simulink model "DPSK_RX"  (R2018a)
settings: Solver=VariableStepAuto  StartTime=0.0  StopTime=inf  RelTol=1e-3
values from neighbouring files (symbols this model uses):
  sdrqpskrx =     [sdrqpskrx.mat]
libraries: commsync2 x3, commrfcorlib x2, dspstat3 x2, commdigbbndpm3 x2, commutil2 x2, sdrublksprivate x1, commrflib2 x1, dspsigops x1, commsequence2 x1, commsink2 x1, dspsrcs4 x1, commfilt2 x1
settings Model: Creator=n53s123  LastModifiedBy=n53s123

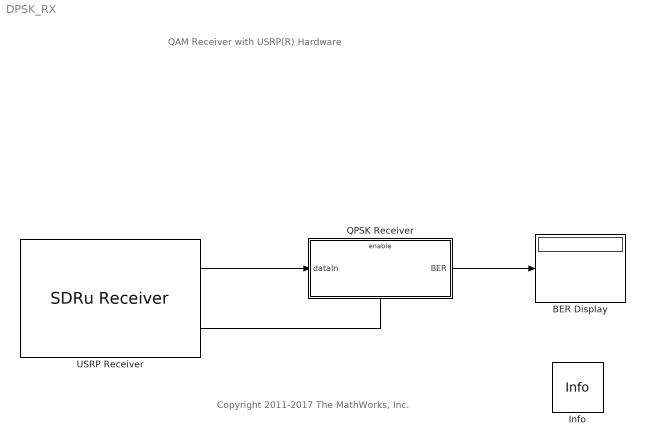
== system DPSK_RX ==
  note: Copyright 2011-2017 The MathWorks, Inc.
  note: QAM Receiver with USRP(R) Hardware
  BER Display : Display
  Info : sdrublksprivate/Info  SystemSampleTime=-1
      settings: SourceProductName=Communications System Toolbox Support Package for USRP(R) Radio  SourceProductBaseCode=USRP
  QPSK Receiver : Subsystem
      mask Display: disp('QAM Receiver')
  USRP Receiver : commsdrhw_v2/SDRu Receiver  SourceLibraryInfo="This block requires <a href=\"http://www.mathworks.com/hardware-support/usrp.html\">Communications System Toolbox Support Package for USRP Radio</a>"  rxtx=rx  initializeIPAddress=0  devMap=0  USRP2_IP=192.168.10.2  USRP_IP_X300=192.168.10.2  USRP_IP_X310=192.168.10.2  USRP_serialNumB200=30B2ACA  USRP_serialNumB210=ECR04ZDBT  platform=N200/N210/USRP2  prevPlatform=N200/N210/USRP2  lastIPAddressPopup=192.168.10.2  USRP_ID=192.168.10.2  LastIPAddress=192.168.10.2  ChannelMapping=1  centerFrequencySrc=Dialog  centerFrequency=15000000  loOffsetSrc=Dialog  loOffset=0  gainSrc=Dialog  gain=0  PPSSource=Internal  clockSource=Internal  masterClkRateParam=100e6  masterClkRateB200=sdrqpskrx.MasterClockRate  masterClkRateB210=sdrqpskrx.MasterClockRate  masterClkRateX300=200e6  masterClkRateX310=200e6  masterClkRate=100e6  decimInterpSrc=Dialog  decimInterp=sdrqpskrx.USRPDecimationFactor  USRP2_IP_NUM=[49 57 50 46 49 54 56 46 49 48 46 50]  TransportDataType=int16  overrunUnderrunPort=off  sampleTime=1/sdrqpskrx.USRPFrontEndSampleRate  outputDatatype=double  frameLength=sdrqpskrx.USRPFrameLength  HOST_DATA_PORT=0  HOST_CONTROL_PORT=0  USRP2_DATA_PORT=0  USRP2_CONTROL_PORT=0  bufferMode=Continuous streaming  EnableBurstMode=off  NumFramesInBurst=100
      settings: SourceProductName=Communications System Toolbox Support Package for USRP(R) Radio  SourceProductBaseCode=USRP
  wires:
  QPSK Receiver/1(BER) -> BER Display/1
  USRP Receiver/2 -> QPSK Receiver/Enable
  USRP Receiver/1 -> QPSK Receiver/1(dataIn)

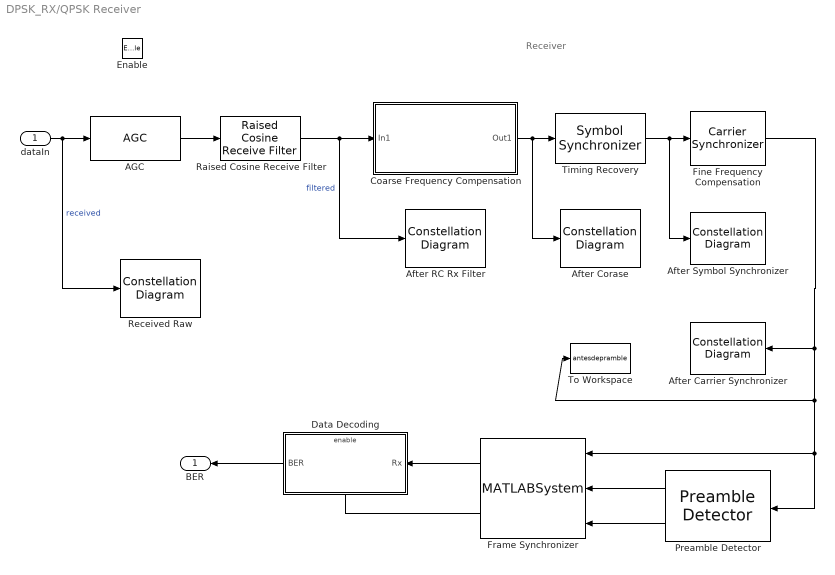
== system DPSK_RX/QPSK Receiver ==
  note: Receiver
  dataIn : Inport
  Enable : EnablePort  PropagateVarSize=During execution
  AGC : commrfcorlib/AGC  LegacyMode=off  DetectorMethod=Rectifier  LoopMethod=Linear  UpdatePeriod=100  StepSize=0.1  AdaptationStepSize=0.01  DesiredOutputPower=sdrqpskrx.DesiredPower  AveragingLength=sdrqpskrx.AveragingLength  MaximumGain=30  MaxPowerGain=sdrqpskrx.MaxPowerGain  GainOutputPort=off  InputPowerOutputPort=off  SimulateUsing=Code generation
      settings: SourceProductName=Communications System Toolbox
  After Carrier Synchronizer : ConstellationDiagram  Tag=ScatterPlot
  After Corase : ConstellationDiagram  Tag=ScatterPlot
  After RC Rx Filter : ConstellationDiagram  Tag=ScatterPlot
  After Symbol Synchronizer : ConstellationDiagram  Tag=ScatterPlot
  Coarse Frequency Compensation : Subsystem
      mask Display: fprintf('Coarse Frequency\nCompensation')
  Data Decoding : Subsystem
      mask Display: disp('Data Decoding');
  Fine Frequency Compensation : commsync2/Carrier Synchronizer  Modulation=QPSK  ModulationPhaseOffset=Auto  CustomPhaseOffset=0  SamplesPerSymbol=sdrqpskrx.Interpolation/sdrqpskrx.Decimation  DampingFactor=1  NormalizedLoopBandwidth=0.01  EstimatedPhaseErrorOutputPort=off  SimulateUsing=Code generation
      settings: SourceProductName=Communications System Toolbox
  Frame Synchronizer : MATLABSystem  System=FrameSynchronizer  Input=Symbol  OutputFrameLength=sdrqpskrx.FrameSize  PreambleLength=sdrqpskrx.BarkerLength  SimulateUsing=Code generation
      mask Type: FrameSynchronizer
      mask Display:
      | disp(['Frame' char(10) 'Synchronizer']);
      | port_label('input',1,'u');
      | port_label('input',2,'idx');
      | port_label('input',3,'dtMt');
      | port_label('output',1,'Frame');
      | port_label('output',2,'Valid');
  Preamble Detector : commsync2/Preamble Detector  Input=Symbol  Preamble=Barker  Threshold=10.5  DetectionMetricOutput=on  Detections=All  SimulateUsing=Code generation
      settings: SourceProductName=Communications System Toolbox  SourceProductBaseCode=CM
  Raised Cosine Receive Filter : commfilt2/Raised Cosine Receive Filter  filtType=Square root  R=sdrqpskrx.RolloffFactor  filtSpan=sdrqpskrx.RaisedCosineFilterSpan  N=sdrqpskrx.Interpolation  downFactor=sdrqpskrx.Decimation  downOffset=0  filterGain=1  InputProcessing=Columns as channels (frame based)  RateOptions=Enforce single-rate processing  framing=Mute  checkCoeff=off  variableName=rcRxFilt  currentFiltSpan=10  D=5  inputOffset=0  sampMode=Mute  saveAsFlag=0  rateMode=Downsampling  checkGain=Normalized  launchFVT=on  roundingMode=Floor  overflowMode=off  coeffDataTypeStr=Inherit: Same word length as input  coeffMin=[]  coeffMax=[]  coeffLastDataTypeStr=Inherit: Same word length as input  accumDataTypeStr=Inherit: Same as product output  accumLastDataTypeStr=Inherit: Same as product output  outputDataTypeStr=Inherit: Same as accumulator  outputMin=[]  outputMax=[]  outputLastDataTypeStr=Inherit: Same as accumulator
  Received Raw : ConstellationDiagram  Tag=ScatterPlot
  Timing Recovery : commsync2/Symbol Synchronizer  Modulation=PAM/PSK/QAM  TimingErrorDetector=Gardner (non-data-aided)  SamplesPerSymbol=2  DampingFactor=1  NormalizedLoopBandwidth=0.01  DetectorGain=sdrqpskrx.TimingErrorDetectorGain  TimingErrorOutputPort=off  SimulateUsing=Code generation
      settings: SourceProductName=Communications System Toolbox  SourceProductBaseCode=CM
  To Workspace : ToWorkspace  VariableName=antesdepramble  SaveFormat=Structure With Time  SampleTime=-1
  BER : Outport
  wires:
  Raised Cosine Receive Filter/1 -> Coarse Frequency Compensation/1(In1), After RC Rx Filter/1  "filtered"
  Preamble Detector/2 -> Frame Synchronizer/3
  Frame Synchronizer/2 -> Data Decoding/Enable
  Preamble Detector/1 -> Frame Synchronizer/2
  Frame Synchronizer/1 -> Data Decoding/1(Rx)
  Coarse Frequency Compensation/1(Out1) -> After Corase/1, Timing Recovery/1
  Data Decoding/1(BER) -> BER/1
  AGC/1 -> Raised Cosine Receive Filter/1
  Fine Frequency Compensation/1 -> To Workspace/1, Frame Synchronizer/1, Preamble Detector/1, After Carrier Synchronizer/1
  Timing Recovery/1 -> Fine Frequency Compensation/1, After Symbol Synchronizer/1
  dataIn/1 -> Received Raw/1, AGC/1  "received"

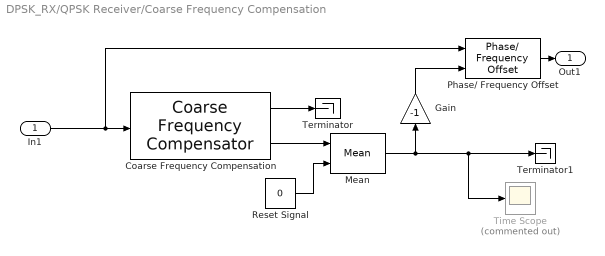
== system DPSK_RX/QPSK Receiver/Coarse Frequency Compensation ==
  In1 : Inport
  Coarse Frequency Compensation : commrfcorlib/Coarse Frequency Compensator  Modulation=QPSK  Algorithm=Correlation-based  FrequencyResolution=25  MaximumFrequencyOffset=12.5e3  SamplesPerSymbol=4  EstimatedFreqOffsetPort=on  SimulateUsing=Code generation
      settings: SourceProductName=Communications System Toolbox  SourceProductBaseCode=CM
  Gain : Gain  Gain=-1
  Mean : dspstat3/Mean  run=on  InputProcessing=Columns as channels (frame based)  reset_popup=Either edge  directionMode=Each column  dimension=1  roiEnable=off  roiType=Rectangles  roiPortion=Entire ROI  roiOutput=Individual statistics for each ROI  roiFlag=off  roundingMode=Floor  overflowMode=off  outputDataTypeStr=Inherit: Same as accumulator  outputMin=[]  outputMax=[]  outputLastDataTypeStr=Inherit: Same as accumulator
  Phase/ Frequency Offset : commrflib2/Phase// Frequency Offset  phaseOffset=0  freqPort=on  freqOffset=0
      settings: SourceProductName=Communications System Toolbox
  Reset Signal : Constant  Value=0
  Terminator : Terminator
  Terminator1 : Terminator
  Time Scope : Scope  Commented=on
  Out1 : Outport
  wires:
  In1/1 -> Phase/ Frequency Offset/1, Coarse Frequency Compensation/1
  Phase/ Frequency Offset/1 -> Out1/1
  Mean/1 -> Time Scope/1, Terminator1/1, Gain/1
  Coarse Frequency Compensation/2 -> Mean/1
  Coarse Frequency Compensation/1 -> Terminator/1
  Gain/1 -> Phase/ Frequency Offset/2
  Reset Signal/1 -> Mean/2

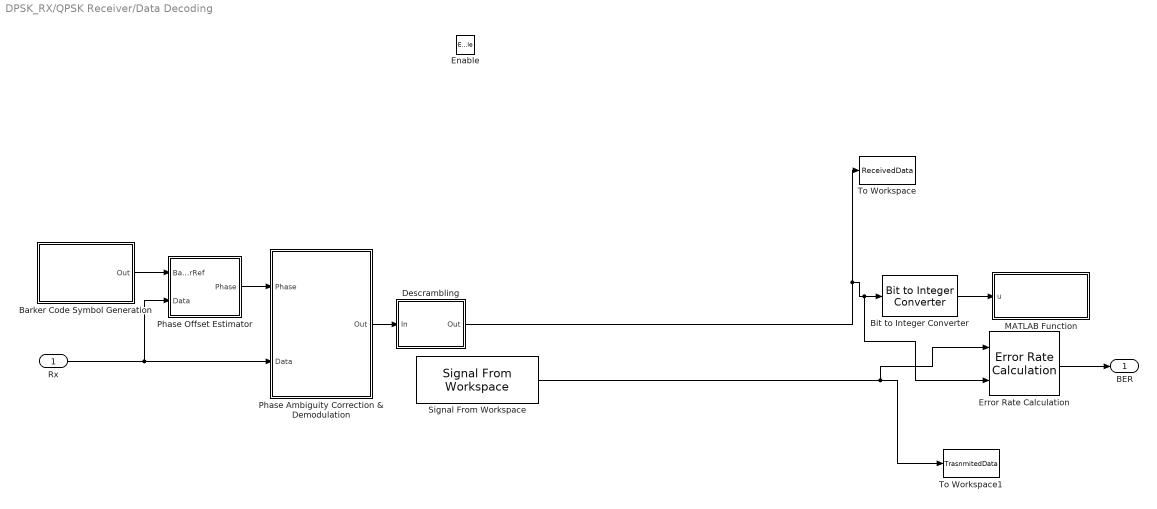
== system DPSK_RX/QPSK Receiver/Data Decoding ==
  Rx : Inport
  Enable : EnablePort
  "Barker Code Symbol Generation " : Subsystem
      mask Display: disp('Barker Code\nSymbol Generation')
  Bit to Integer Converter : commutil2/Bit to Integer Converter  nbits=7  bitOrder=MSB first  signedOutputValues=Unsigned  outDtype=Inherit via internal rule  outDtypeSigned=Inherit via internal rule
  Descrambling : Subsystem
      mask Display: disp('Descrambling');
  Error Rate Calculation : commsink2/Error Rate Calculation  N=0  st_delay=0  cp_mode=Select samples from mask  subframe=sdrqpskrx.BerMask  PMode=Port  WsName=ErrorVec  RsMode2=off  stop=off  numErr=100  maxBits=1e6
  MATLAB Function : MATLAB Function  TreatAsAtomicUnit=on
  Phase Ambiguity Correction & Demodulation : Subsystem
      mask Display: disp('Phase Ambiguity\nCorrection\n& Demodulation');
  Phase Offset Estimator : Subsystem
  Signal From Workspace : dspsrcs4/Signal From Workspace  X=sdrqpskrx.MessageBits  Ts=1/sdrqpskrx.PayloadLength*sdrqpskrx.FrameTime  nsamps=sdrqpskrx.MessageLength * 7 * sdrqpskrx.NumberOfMessage  OutputAfterFinalValue=Cyclic repetition  ignoreOrWarnInputAndFrameLengths=off  OutputFrames=off
  To Workspace : ToWorkspace  VariableName=ReceivedData  SampleTime=-1
  To Workspace1 : ToWorkspace  VariableName=TrasnmitedData  SampleTime=-1
  BER : Outport
  wires:
  "Barker Code Symbol Generation "/1(Out) -> Phase Offset Estimator/1(BarkerRef)
  Phase Offset Estimator/1(Phase) -> Phase Ambiguity Correction & Demodulation/1(Phase)
  Rx/1 -> Phase Offset Estimator/2(Data), Phase Ambiguity Correction & Demodulation/2(Data)
  Error Rate Calculation/1 -> BER/1
  Phase Ambiguity Correction & Demodulation/1(Out) -> Descrambling/1(In)
  Signal From Workspace/1 -> Error Rate Calculation/1, To Workspace1/1
  Bit to Integer Converter/1 -> MATLAB Function/1(u)
  Descrambling/1(Out) -> Error Rate Calculation/2, Bit to Integer Converter/1, To Workspace/1

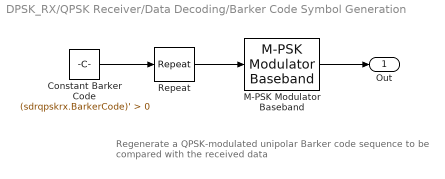
== system DPSK_RX/QPSK Receiver/Data Decoding/Barker Code Symbol Generation  ==
  note: Regenerate a QPSK-modulated unipolar Barker code sequence
      | to be compared with the received data
  Constant Barker Code : Constant  Value=(sdrqpskrx.BarkerCode)' > 0  VectorParams1D=off  OutDataTypeStr=double
  M-PSK Modulator Baseband : commdigbbndpm3/M-PSK Modulator Baseband  M=16  InType=Bit  Enc=Gray  Mapping=[0:7]  Ph=0  outDtype=double  outWordLen=16  outUDDataType=sfix(16)  outFracLenMode=Best precision  outFracLen=15  outDataTypeStr=double  outLastDataTypeStr=double
      settings: SourceProductName=Communications System Toolbox
  Repeat : dspsigops/Repeat  N=4  InputProcessing=Columns as channels (frame based)  RateOptions=Enforce single-rate processing  ic=0  mode=Unused parameter value
      settings: SourceProductName=DSP System Toolbox
  Out : Outport
  wires:
  Constant Barker Code/1 -> Repeat/1
  Repeat/1 -> M-PSK Modulator Baseband/1
  M-PSK Modulator Baseband/1 -> Out/1

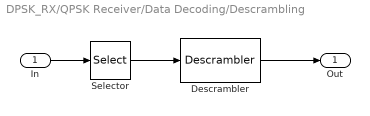
== system DPSK_RX/QPSK Receiver/Data Decoding/Descrambling ==
  In : Inport
  Descrambler : commsequence2/Descrambler  M=2  poly=[1 1 1 0 1]  iniStaSource=Dialog Parameter  ini_sta=[0 0 0 0]  resetViaPort=off
      settings: SourceProductName=Communications System Toolbox  SourceProductBaseCode=CM
  Selector : Selector  IndexOptions=Index vector (dialog)  Indices=[sdrqpskrx.HeaderLength+(1 : sdrqpskrx.PayloadLength)]  OutputSizes=1
  Out : Outport
  wires:
  In/1 -> Selector/1
  Selector/1 -> Descrambler/1
  Descrambler/1 -> Out/1

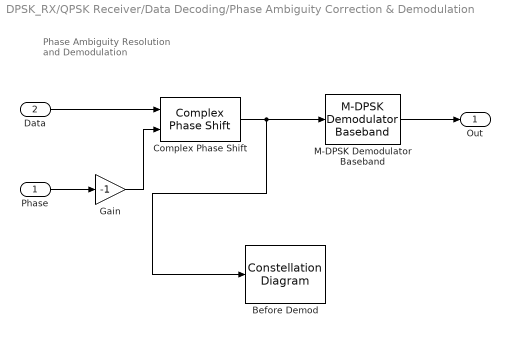
== system DPSK_RX/QPSK Receiver/Data Decoding/Phase Ambiguity Correction & Demodulation ==
  note: Phase Ambiguity Resolution
      | and Demodulation
  Phase : Inport
  Data : Inport  Port=2
  "Before Demod " : ConstellationDiagram  Tag=ScatterPlot
  Complex Phase Shift : commutil2/Complex Phase Shift
      settings: SourceProductName=Communications System Toolbox  SourceProductBaseCode=CM
  Gain : Gain  Gain=-1  OutDataTypeStr=Inherit: Same as input
  M-DPSK Demodulator Baseband : commdigbbndpm3/M-DPSK Demodulator Baseband  M=16  OutType=Bit  Dec=Gray  Ph=0  outDtype1=Inherit via internal rule  outDtype2=Inherit via internal rule
      settings: SourceProductName=Communications System Toolbox  SourceProductBaseCode=CM
  Out : Outport
  wires:
  Phase/1 -> Gain/1
  M-DPSK Demodulator Baseband/1 -> Out/1
  Data/1 -> Complex Phase Shift/1
  Gain/1 -> Complex Phase Shift/2
  Complex Phase Shift/1 -> M-DPSK Demodulator Baseband/1, "Before Demod "/1

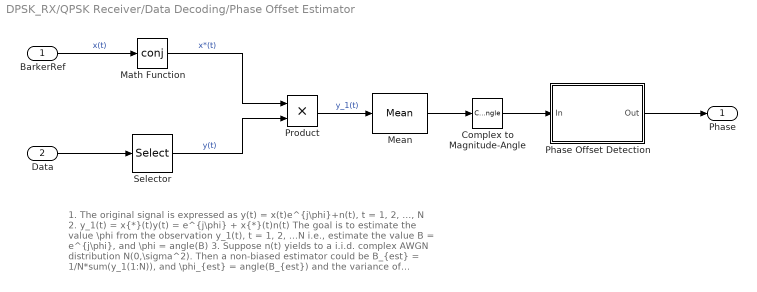
== system DPSK_RX/QPSK Receiver/Data Decoding/Phase Offset Estimator ==
  note: 1. The original signal is expressed as y(t) = x(t)e^{j\phi}+n(t), t = 1, 2, ..., N
      | 2. y_1(t) = x{*}(t)y(t) = e^{j\phi} + x{*}(t)n(t)
      | The goal is to estimate the value \phi from the observation y_1(t), t = 1, 2, ...N
      | i.e., estimate the value B = e^{j\phi}, and \phi = angle(B)
      | 3. Suppose n(t) yields to a i.i.d. complex AWGN distribution N(0,\sigma^2).
      | Then a non-biased estimator could be
      | B_{est} = 1/N*sum(y_1(1:N)), and \phi_{est} = angle(B_{est})
      | and the variance of B_{est} is \sigma^2/N
  BarkerRef : Inport
  Data : Inport  Port=2
  Complex to Magnitude-Angle : ComplexToMagnitudeAngle  Output=Angle
  Math Function : Math  Operator=conj  SaturateOnIntegerOverflow=on
  Mean : dspstat3/Mean  run=off  InputProcessing=Columns as channels (frame based)  reset_popup=None  directionMode=Each column  dimension=1  roiEnable=off  roiType=Rectangles  roiPortion=Entire ROI  roiOutput=Individual statistics for each ROI  roiFlag=off  roundingMode=Floor  overflowMode=off  outputDataTypeStr=Inherit: Same as accumulator  outputMin=[]  outputMax=[]  outputLastDataTypeStr=Inherit: Same as accumulator
  Phase Offset Detection : MATLAB Function  TreatAsAtomicUnit=on
  Product : Product  RndMeth=Zero
  Selector : Selector  IndexOptions=Index vector (dialog)  Indices=[1:sdrqpskrx.BarkerLength]  OutputSizes=1
  Phase : Outport
  wires:
  Data/1 -> Selector/1
  BarkerRef/1 -> Math Function/1  "x(t)"
  Selector/1 -> Product/2  "y(t)"
  Math Function/1 -> Product/1  "x*(t)"
  Product/1 -> Mean/1  "y_1(t)"
  Mean/1 -> Complex to Magnitude-Angle/1
  Complex to Magnitude-Angle/1 -> Phase Offset Detection/1(In)
  Phase Offset Detection/1(Out) -> Phase/1

== matlab function DPSK_RX/QPSK Receiver/Data Decoding/MATLAB Function ==
  data: u input
function IntegerToASCII(u)
fprintf('%s', char(u'));
end

== matlab function DPSK_RX/QPSK Receiver/Data Decoding/Phase Offset Estimator/Phase Offset Detection ==
  data: In input; Out output
function Out = phasedecision(In)
% Map the estimated phase to one of -pi, -pi/2, 0, pi/2,  
%#codegen
Out = round(In.*2./pi)./2.*pi;
% The above processing is equivalent to the following processing using
% if/else statements
%
% if In<pi/4 && In>-pi/4
%     Out = 0;
% elseif In>=pi/4 && In<pi*3/4
%     Out = pi/2;
% elseif In>=pi*3/4 || In<=-pi*3/4
%     Out = -pi;
% else
%     Out = -pi/2;
% end
